simulink model "MFTiresLongitudinalSSC"  (R2026b)
settings: Solver=VariableStepAuto
undefined symbols (not defined in the file): AxlFL, AxlFR, AxlRL, AxlRR, PlntWhlDampCoeffFrnt, PlntWhlDampCoeffRear, PlntWhlLdRadius
libraries: fl_lib x16, nesl_utility_internal x10, sdl_lib x4
settings Model: Creator=The MathWorks, Inc.  LastModifiedBy=The MathWorks, Inc.
settings OptimizationCC: ReuseModelBlockBuffer=off
settings DebuggingCC: SubsystemReferenceDiagnosticForUnitTest=warning
settings SimscapeCC: SimscapeUseEnergyAccounting=off

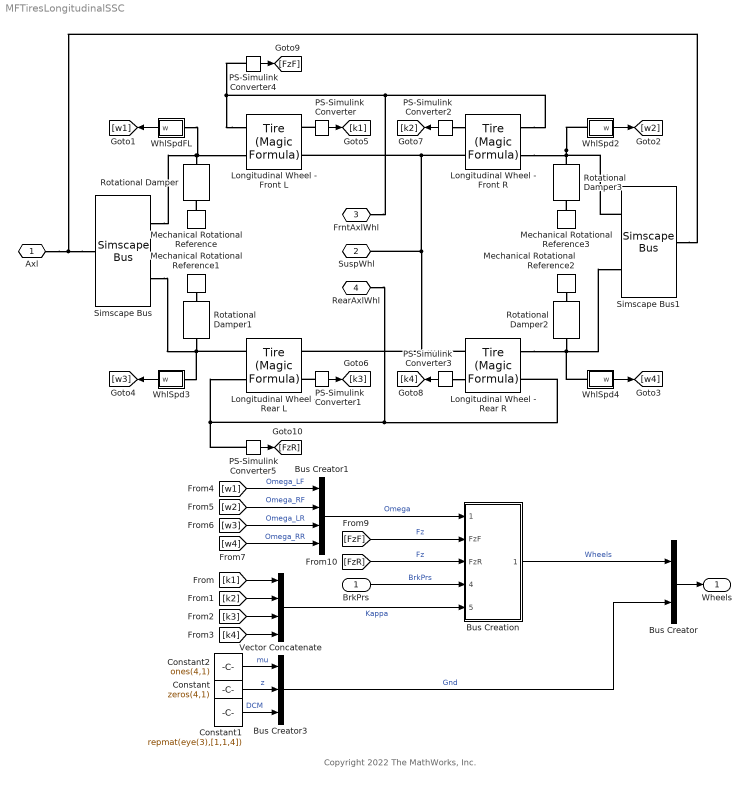
== system MFTiresLongitudinalSSC ==
  note: Copyright 2022 The MathWorks, Inc.
  BrkPrs : Inport
  Bus Creator : BusCreator  Inputs=2
  Bus Creator1 : BusCreator  Inputs=4
  Bus Creator3 : BusCreator  Inputs=3
  Bus Creation : Subsystem
  Constant : Constant  Value=zeros(4,1)  SampleTime=-1
  Constant1 : Constant  Value=repmat(eye(3),[1,1,4])  SampleTime=-1
  Constant2 : Constant  Value=ones(4,1)  SampleTime=-1
  Longitudinal Wheel - Front L : sdl_lib/Tires & Vehicles/Tire (Magic Formula)  parameterization=sdl.enum.magic_tire_model.constant  F_z1=3000 N  F_x1=3500 N  kappa1=10  B_m=PlntWhlLongStfFctr  C_m=PlntWhlLongShapeFctr  D_m=PlntWhlLongPeakFctr  E_m=PlntWhlLongCuvFctr  fz0=4000 N  p_Cx=1.685  p_Dx=[1.21, -.037]  p_Ex=[.344, .095, -.02, 0]  p_Kx=[21.51, -.163, .245]  p_Hx=[-.002, .002]  p_Vx=[0, 0]  rolling_radius_model=sdl.enum.RollingRadiusParameterization.Constant  r_e=PlntWhlLdRadius m  r_0=0.3 m  breff=8.39  dreff=0.26  freff=0.074  q_re0=0.99  q_v1=0.008  longvl=17 m/s  cz=5e5 N/m  model_resistance=simscape.enum.onoff.on  resistance_model=sdl.enum.rollingResistanceParameterization.velocity  coeff=0.015  p_tire=PlntWhlPrsFrnt Pa  alpha=PlntWhlTirPrsExp  beta=PlntWhlNrmlForceExp  coeff_a=PlntWhlVelIndpntForceCff  coeff_b=PlntWhlLnrVelForceComp s/m  coeff_c=PlntWhlQuadVelForceComp s^2/m^2  p_tire0=240e3 Pa  fz0_resistance=4000 N  vH0=16 m/s  q_Sy=[.0082, 0, .0014, .001, 0, 0, 1.08, -.5]  v_thr=PlntWhlRollResVelThresh m/s  enable_scaling_coefficients=false  lfzO=1  lcx=1  lmux=1  lex=1  lkx=1  lhx=1  lvx=1  lmy=1  model_compliance=sdl.enum.compliance.off  stiffness=PlntWhlCompStiff N/m  damping=PlntWhlCompDamp N*s/m  model_inertia=sdl.enum.model_inertia.on  inertia=PlntWhlInertiaFrnt kg*m^2  initial_velocity=0 rad/s  vxlow=1 m/s  v_tr_thr=PlntWhlVelThresh m/s  kpumin=PlntWhlMinSlipRatio  kpumax=PlntWhlMaxSlipRatio
  Longitudinal Wheel - Front R : sdl_lib/Tires & Vehicles/Tire (Magic Formula)  parameterization=sdl.enum.magic_tire_model.constant  F_z1=3000 N  F_x1=3500 N  kappa1=10  B_m=PlntWhlLongStfFctr  C_m=PlntWhlLongShapeFctr  D_m=PlntWhlLongPeakFctr  E_m=PlntWhlLongCuvFctr  fz0=4000 N  p_Cx=1.685  p_Dx=[1.21, -.037]  p_Ex=[.344, .095, -.02, 0]  p_Kx=[21.51, -.163, .245]  p_Hx=[-.002, .002]  p_Vx=[0, 0]  rolling_radius_model=sdl.enum.RollingRadiusParameterization.Constant  r_e=PlntWhlLdRadius m  r_0=0.3 m  breff=8.39  dreff=0.26  freff=0.074  q_re0=0.99  q_v1=0.008  longvl=17 m/s  cz=5e5 N/m  model_resistance=simscape.enum.onoff.on  resistance_model=sdl.enum.rollingResistanceParameterization.velocity  coeff=0.015  p_tire=PlntWhlPrsFrnt Pa  alpha=PlntWhlTirPrsExp  beta=PlntWhlNrmlForceExp  coeff_a=PlntWhlVelIndpntForceCff  coeff_b=PlntWhlLnrVelForceComp s/m  coeff_c=PlntWhlQuadVelForceComp s^2/m^2  p_tire0=240e3 Pa  fz0_resistance=4000 N  vH0=16 m/s  q_Sy=[.0082, 0, .0014, .001, 0, 0, 1.08, -.5]  v_thr=PlntWhlRollResVelThresh m/s  enable_scaling_coefficients=false  lfzO=1  lcx=1  lmux=1  lex=1  lkx=1  lhx=1  lvx=1  lmy=1  model_compliance=sdl.enum.compliance.off  stiffness=PlntWhlCompStiff N/m  damping=PlntWhlCompDamp N*s/m  model_inertia=sdl.enum.model_inertia.on  inertia=PlntWhlInertiaFrnt kg*m^2  initial_velocity=0 rad/s  vxlow=1 m/s  v_tr_thr=PlntWhlVelThresh m/s  kpumin=PlntWhlMinSlipRatio  kpumax=PlntWhlMaxSlipRatio
  Longitudinal Wheel - Rear L : sdl_lib/Tires & Vehicles/Tire (Magic Formula)  parameterization=sdl.enum.magic_tire_model.constant  F_z1=3000 N  F_x1=3500 N  kappa1=10  B_m=PlntWhlLongStfFctr  C_m=PlntWhlLongShapeFctr  D_m=PlntWhlLongPeakFctr  E_m=PlntWhlLongCuvFctr  fz0=4000 N  p_Cx=1.685  p_Dx=[1.21, -.037]  p_Ex=[.344, .095, -.02, 0]  p_Kx=[21.51, -.163, .245]  p_Hx=[-.002, .002]  p_Vx=[0, 0]  rolling_radius_model=sdl.enum.RollingRadiusParameterization.Constant  r_e=PlntWhlLdRadius m  r_0=0.3 m  breff=8.39  dreff=0.26  freff=0.074  q_re0=0.99  q_v1=0.008  longvl=17 m/s  cz=5e5 N/m  model_resistance=simscape.enum.onoff.on  resistance_model=sdl.enum.rollingResistanceParameterization.velocity  coeff=0.015  p_tire=PlntWhlPrsRear Pa  alpha=PlntWhlTirPrsExp  beta=PlntWhlNrmlForceExp  coeff_a=PlntWhlVelIndpntForceCff  coeff_b=PlntWhlLnrVelForceComp s/m  coeff_c=PlntWhlQuadVelForceComp s^2/m^2  p_tire0=240e3 Pa  fz0_resistance=4000 N  vH0=16 m/s  q_Sy=[.0082, 0, .0014, .001, 0, 0, 1.08, -.5]  v_thr=PlntWhlRollResVelThresh m/s  enable_scaling_coefficients=false  lfzO=1  lcx=1  lmux=1  lex=1  lkx=1  lhx=1  lvx=1  lmy=1  model_compliance=sdl.enum.compliance.off  stiffness=PlntWhlCompStiff N/m  damping=PlntWhlCompDamp N*s/m  model_inertia=sdl.enum.model_inertia.on  inertia=PlntWhlInertiaRear kg*m^2  initial_velocity=0 rad/s  vxlow=1 m/s  v_tr_thr=PlntWhlVelThresh m/s  kpumin=PlntWhlMinSlipRatio  kpumax=PlntWhlMaxSlipRatio
  Longitudinal Wheel - Rear R : sdl_lib/Tires & Vehicles/Tire (Magic Formula)  parameterization=sdl.enum.magic_tire_model.constant  F_z1=3000 N  F_x1=3500 N  kappa1=10  B_m=PlntWhlLongStfFctr  C_m=PlntWhlLongShapeFctr  D_m=PlntWhlLongPeakFctr  E_m=PlntWhlLongCuvFctr  fz0=4000 N  p_Cx=1.685  p_Dx=[1.21, -.037]  p_Ex=[.344, .095, -.02, 0]  p_Kx=[21.51, -.163, .245]  p_Hx=[-.002, .002]  p_Vx=[0, 0]  rolling_radius_model=sdl.enum.RollingRadiusParameterization.Constant  r_e=PlntWhlLdRadius m  r_0=0.3 m  breff=8.39  dreff=0.26  freff=0.074  q_re0=0.99  q_v1=0.008  longvl=17 m/s  cz=5e5 N/m  model_resistance=simscape.enum.onoff.on  resistance_model=sdl.enum.rollingResistanceParameterization.velocity  coeff=0.015  p_tire=PlntWhlPrsRear Pa  alpha=PlntWhlTirPrsExp  beta=PlntWhlNrmlForceExp  coeff_a=PlntWhlVelIndpntForceCff  coeff_b=PlntWhlLnrVelForceComp s/m  coeff_c=PlntWhlQuadVelForceComp s^2/m^2  p_tire0=240e3 Pa  fz0_resistance=4000 N  vH0=16 m/s  q_Sy=[.0082, 0, .0014, .001, 0, 0, 1.08, -.5]  v_thr=PlntWhlRollResVelThresh m/s  enable_scaling_coefficients=false  lfzO=1  lcx=1  lmux=1  lex=1  lkx=1  lhx=1  lvx=1  lmy=1  model_compliance=sdl.enum.compliance.off  stiffness=PlntWhlCompStiff N/m  damping=PlntWhlCompDamp N*s/m  model_inertia=sdl.enum.model_inertia.on  inertia=PlntWhlInertiaRear kg*m^2  initial_velocity=0 rad/s  vxlow=1 m/s  v_tr_thr=PlntWhlVelThresh m/s  kpumin=PlntWhlMinSlipRatio  kpumax=PlntWhlMaxSlipRatio
  Mechanical Rotational Reference{,1..3} (4 alike) : fl_lib/Mechanical/Rotational Elements/Mechanical Rotational Reference
  PS-Simulink Converter{,1..5} (6 alike) : nesl_utility_internal/PS-Simulink Converter  PhysicalDomain=network_engine_domain  SubClassName=ps_output  LeftPortType=input  RightPortType=output  PseudoPeriodic=off  Frequencies=[]  VectorFormat=inherit  Unit=inherit  AffineConversion=off
  Rotational Damper : fl_lib/Mechanical/Rotational Elements/Rotational Damper  D=PlntWhlDampCoeffFrnt N*m*s/rad  w_specify=off  w_priority=None  w=0 rad/s  w_nominal_specify=off  w_nominal_value=1  w_nominal_unit=rad/s  t_specify=off  t_priority=None  t=0 N*m  t_nominal_specify=off  t_nominal_value=1  t_nominal_unit=N*m
  Rotational Damper1 : fl_lib/Mechanical/Rotational Elements/Rotational Damper  D=PlntWhlDampCoeffRear N*m*s/rad  w_specify=off  w_priority=None  w=0 rad/s  w_nominal_specify=off  w_nominal_value=1  w_nominal_unit=rad/s  t_specify=off  t_priority=None  t=0 N*m  t_nominal_specify=off  t_nominal_value=1  t_nominal_unit=N*m
  Rotational Damper2 : fl_lib/Mechanical/Rotational Elements/Rotational Damper  D=PlntWhlDampCoeffRear N*m*s/rad  w_specify=off  w_priority=None  w=0 rad/s  w_nominal_specify=off  w_nominal_value=1  w_nominal_unit=rad/s  t_specify=off  t_priority=None  t=0 N*m  t_nominal_specify=off  t_nominal_value=1  t_nominal_unit=N*m
  Rotational Damper3 : fl_lib/Mechanical/Rotational Elements/Rotational Damper  D=PlntWhlDampCoeffFrnt N*m*s/rad  w_specify=off  w_priority=None  w=0 rad/s  w_nominal_specify=off  w_nominal_value=1  w_nominal_unit=rad/s  t_specify=off  t_priority=None  t=0 N*m  t_nominal_specify=off  t_nominal_value=1  t_nominal_unit=N*m
  Simscape Bus : SimscapeBus  HierarchyStrings=AxlFL;AxlRL
  Simscape Bus1 : SimscapeBus  HierarchyStrings=AxlFR;AxlRR
  Vector Concatenate : Concatenate  NumInputs=4
  WhlSpd2 : Subsystem
  WhlSpd3 : Subsystem
  WhlSpd4 : Subsystem
  WhlSpdFL : Subsystem
  Axl : PMIOPort  Side=Left
  SuspWhl : PMIOPort  Port=2  Side=Left
  FrntAxlWhl : PMIOPort  Port=3  Side=Left
  RearAxlWhl : PMIOPort  Port=4  Side=Left
  Wheels : Outport
  wires:
  PS-Simulink Converter5/1 -> [FzR]
  [FzF] -> Bus Creation/2(FzF)  "Fz"
  PS-Simulink Converter4/1 -> [FzF]
  WhlSpdFL/1(w) -> [w1]
  [w1] -> Bus Creator1/1  "Omega_LF"
  BrkPrs/1 -> Bus Creation/4(BrkPrs)  "BrkPrs"
  [w3] -> Bus Creator1/3  "Omega_LR"
  PS-Simulink Converter1/1 -> [k3]
  WhlSpd3/1(w) -> [w3]
  [k4] -> Vector Concatenate/4
  PS-Simulink Converter/1 -> [k1]
  [w2] -> Bus Creator1/2  "Omega_RF"
  [FzR] -> Bus Creation/3(FzR)  "Fz"
  [w4] -> Bus Creator1/4  "Omega_RR"
  Bus Creator1/1 -> Bus Creation/1(Omega)  "Omega"
  PS-Simulink Converter2/1 -> [k2]
  WhlSpd4/1(w) -> [w4]
  Vector Concatenate/1 -> Bus Creation/5(Kappa)  "Kappa"
  PS-Simulink Converter3/1 -> [k4]
  [k1] -> Vector Concatenate/1
  WhlSpd2/1(w) -> [w2]
  [k3] -> Vector Concatenate/3
  [k2] -> Vector Concatenate/2
  Bus Creation/1(Wheels) -> Bus Creator/1  "Wheels"
  Constant2/1 -> Bus Creator3/1  "mu"
  Constant/1 -> Bus Creator3/2  "z"
  Constant1/1 -> Bus Creator3/3  "DCM"
  Bus Creator3/1 -> Bus Creator/2  "Gnd"
  Bus Creator/1 -> Wheels/1
  connections:
  RearAxlWhl/RConn1 -- PS-Simulink Converter5/LConn1 -- Longitudinal Wheel - Rear L/LConn1 -- Longitudinal Wheel - Rear R/LConn1
  WhlSpdFL/LConn1 -- Rotational Damper/LConn1 -- Simscape Bus/LConn1 -- Longitudinal Wheel - Front L/LConn2
  Rotational Damper2/LConn1 -- WhlSpd4/LConn1 -- Longitudinal Wheel - Rear R/LConn2 -- Simscape Bus1/LConn2
  Longitudinal Wheel - Front L/LConn1 -- Longitudinal Wheel - Front R/LConn1 -- FrntAxlWhl/RConn1 -- PS-Simulink Converter4/LConn1
  Simscape Bus/RConn1 -- Simscape Bus1/RConn1 -- Axl/RConn1
  Longitudinal Wheel - Rear L/LConn2 -- WhlSpd3/LConn1 -- Simscape Bus/LConn2 -- Rotational Damper1/LConn1
  Simscape Bus1/LConn1 -- WhlSpd2/LConn1 -- Rotational Damper3/LConn1 -- Longitudinal Wheel - Front R/LConn2
  Longitudinal Wheel - Rear R/RConn2 -- Longitudinal Wheel - Front R/RConn2 -- Longitudinal Wheel - Front L/RConn2 -- SuspWhl/RConn1 -- Longitudinal Wheel - Rear L/RConn2
  PS-Simulink Converter1/LConn1 -- Longitudinal Wheel - Rear L/RConn1
  Mechanical Rotational Reference1/LConn1 -- Rotational Damper1/RConn1
  Mechanical Rotational Reference2/LConn1 -- Rotational Damper2/RConn1
  Mechanical Rotational Reference/LConn1 -- Rotational Damper/RConn1
  PS-Simulink Converter3/LConn1 -- Longitudinal Wheel - Rear R/RConn1
  Mechanical Rotational Reference3/LConn1 -- Rotational Damper3/RConn1
  PS-Simulink Converter/LConn1 -- Longitudinal Wheel - Front L/RConn1
  PS-Simulink Converter2/LConn1 -- Longitudinal Wheel - Front R/RConn1

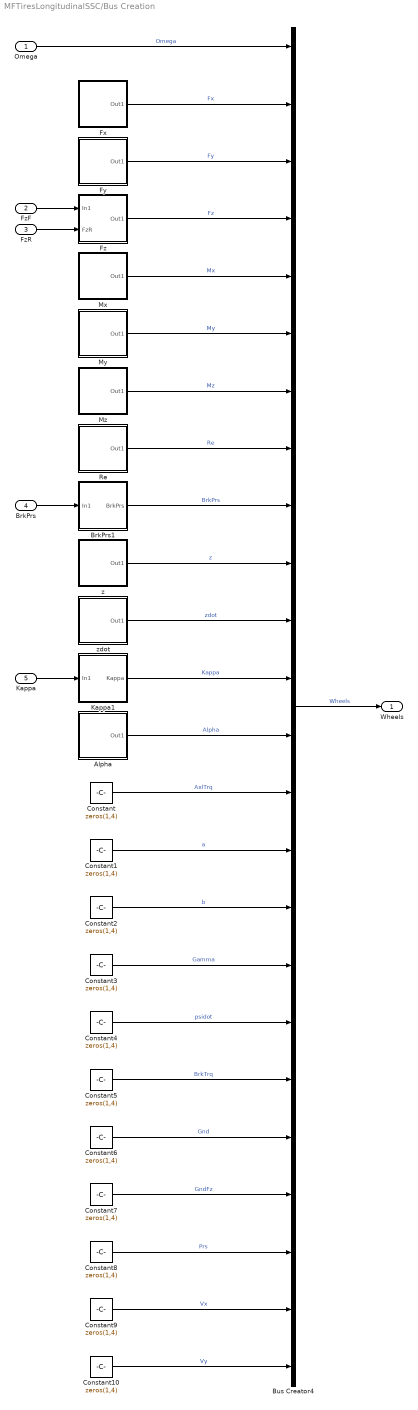
== system MFTiresLongitudinalSSC/Bus Creation ==
  Omega : Inport
  FzF : Inport  Port=2
  FzR : Inport  Port=3
  BrkPrs : Inport  Port=4
  Kappa : Inport  Port=5
  Alpha : Subsystem
  BrkPrs1 : Subsystem
  Bus Creator4 : BusCreator  Inputs=24
  Constant{,1..10} (11 alike) : Constant  Value=zeros(1,4)  SampleTime=-1
  Fx : Subsystem
  Fy : Subsystem
  Fz : Subsystem
  Kappa1 : Subsystem
  Mx : Subsystem
  My : Subsystem
  Mz : Subsystem
  Re : Subsystem
  z : Subsystem
  zdot : Subsystem
  Wheels : Outport
  wires:
  BrkPrs1/1(BrkPrs) -> Bus Creator4/9  "BrkPrs"
  Bus Creator4/1 -> Wheels/1  "Wheels"
  Alpha/1(Out1) -> Bus Creator4/13  "Alpha"
  My/1(Out1) -> Bus Creator4/6  "My"
  Fy/1(Out1) -> Bus Creator4/3  "Fy"
  z/1(Out1) -> Bus Creator4/10  "z"
  Omega/1 -> Bus Creator4/1  "Omega"
  Mz/1(Out1) -> Bus Creator4/7  "Mz"
  Kappa1/1(Kappa) -> Bus Creator4/12  "Kappa"
  zdot/1(Out1) -> Bus Creator4/11  "zdot"
  Mx/1(Out1) -> Bus Creator4/5  "Mx"
  Fx/1(Out1) -> Bus Creator4/2  "Fx"
  Fz/1(Out1) -> Bus Creator4/4  "Fz"
  Re/1(Out1) -> Bus Creator4/8  "Re"
  FzF/1 -> Fz/1(In1)
  FzR/1 -> Fz/2(FzR)
  BrkPrs/1 -> BrkPrs1/1(In1)
  Kappa/1 -> Kappa1/1(In1)
  Constant/1 -> Bus Creator4/14  "AxlTrq"
  Constant1/1 -> Bus Creator4/15  "a"
  Constant2/1 -> Bus Creator4/16  "b"
  Constant3/1 -> Bus Creator4/17  "Gamma"
  Constant4/1 -> Bus Creator4/18  "psidot"
  Constant5/1 -> Bus Creator4/19  "BrkTrq"
  Constant6/1 -> Bus Creator4/20  "Gnd"
  Constant7/1 -> Bus Creator4/21  "GndFz"
  Constant8/1 -> Bus Creator4/22  "Prs"
  Constant9/1 -> Bus Creator4/23  "Vx"
  Constant10/1 -> Bus Creator4/24  "Vy"

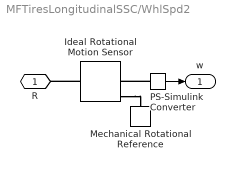
== system MFTiresLongitudinalSSC/WhlSpd2 ==
  Ideal Rotational Motion Sensor : fl_lib/Mechanical/Mechanical Sensors/Ideal Rotational Motion Sensor  reference=foundation.enum.MeasurementReference.difference  acceleration_port=false  velocity_port=true  position_port=true  wrap_angle=simscape.enum.onoff.off  offset=0 rad
  Mechanical Rotational Reference : fl_lib/Mechanical/Rotational Elements/Mechanical Rotational Reference
  PS-Simulink Converter : nesl_utility_internal/PS-Simulink Converter  PhysicalDomain=network_engine_domain  SubClassName=ps_output  LeftPortType=input  RightPortType=output  PseudoPeriodic=off  Frequencies=[]  VectorFormat=inherit  Unit=inherit  AffineConversion=off
  R : PMIOPort  Side=Left
  w : Outport
  wires:
  PS-Simulink Converter/1 -> w/1
  connections:
  PS-Simulink Converter/LConn1 -- Ideal Rotational Motion Sensor/RConn2
  Ideal Rotational Motion Sensor/LConn1 -- R/RConn1
  Ideal Rotational Motion Sensor/RConn1 -- Mechanical Rotational Reference/LConn1

== system MFTiresLongitudinalSSC/WhlSpd3 ==
  Ideal Rotational Motion Sensor : fl_lib/Mechanical/Mechanical Sensors/Ideal Rotational Motion Sensor  reference=foundation.enum.MeasurementReference.difference  acceleration_port=false  velocity_port=true  position_port=true  wrap_angle=simscape.enum.onoff.off  offset=0 rad
  Mechanical Rotational Reference : fl_lib/Mechanical/Rotational Elements/Mechanical Rotational Reference
  PS-Simulink Converter : nesl_utility_internal/PS-Simulink Converter  PhysicalDomain=network_engine_domain  SubClassName=ps_output  LeftPortType=input  RightPortType=output  PseudoPeriodic=off  Frequencies=[]  VectorFormat=inherit  Unit=inherit  AffineConversion=off
  R : PMIOPort  Side=Left
  w : Outport
  wires:
  PS-Simulink Converter/1 -> w/1
  connections:
  PS-Simulink Converter/LConn1 -- Ideal Rotational Motion Sensor/RConn2
  Ideal Rotational Motion Sensor/LConn1 -- R/RConn1
  Ideal Rotational Motion Sensor/RConn1 -- Mechanical Rotational Reference/LConn1

== system MFTiresLongitudinalSSC/WhlSpd4 ==
  Ideal Rotational Motion Sensor : fl_lib/Mechanical/Mechanical Sensors/Ideal Rotational Motion Sensor  reference=foundation.enum.MeasurementReference.difference  acceleration_port=false  velocity_port=true  position_port=true  wrap_angle=simscape.enum.onoff.off  offset=0 rad
  Mechanical Rotational Reference : fl_lib/Mechanical/Rotational Elements/Mechanical Rotational Reference
  PS-Simulink Converter : nesl_utility_internal/PS-Simulink Converter  PhysicalDomain=network_engine_domain  SubClassName=ps_output  LeftPortType=input  RightPortType=output  PseudoPeriodic=off  Frequencies=[]  VectorFormat=inherit  Unit=inherit  AffineConversion=off
  R : PMIOPort  Side=Left
  w : Outport
  wires:
  PS-Simulink Converter/1 -> w/1
  connections:
  Ideal Rotational Motion Sensor/RConn1 -- Mechanical Rotational Reference/LConn1
  Ideal Rotational Motion Sensor/LConn1 -- R/RConn1
  PS-Simulink Converter/LConn1 -- Ideal Rotational Motion Sensor/RConn2

== system MFTiresLongitudinalSSC/WhlSpdFL ==
  Ideal Rotational Motion Sensor : fl_lib/Mechanical/Mechanical Sensors/Ideal Rotational Motion Sensor  reference=foundation.enum.MeasurementReference.difference  acceleration_port=false  velocity_port=true  position_port=true  wrap_angle=simscape.enum.onoff.off  offset=0 rad
  Mechanical Rotational Reference : fl_lib/Mechanical/Rotational Elements/Mechanical Rotational Reference
  PS-Simulink Converter : nesl_utility_internal/PS-Simulink Converter  PhysicalDomain=network_engine_domain  SubClassName=ps_output  LeftPortType=input  RightPortType=output  PseudoPeriodic=off  Frequencies=[]  VectorFormat=inherit  Unit=inherit  AffineConversion=off
  R : PMIOPort  Side=Left
  w : Outport
  wires:
  PS-Simulink Converter/1 -> w/1
  connections:
  Ideal Rotational Motion Sensor/RConn1 -- Mechanical Rotational Reference/LConn1
  Ideal Rotational Motion Sensor/LConn1 -- R/RConn1
  PS-Simulink Converter/LConn1 -- Ideal Rotational Motion Sensor/RConn2

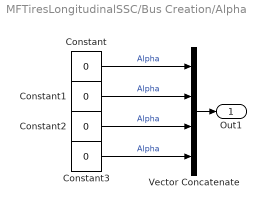
== system MFTiresLongitudinalSSC/Bus Creation/Alpha ==
  Constant{,1..3} (4 alike) : Constant  Value=0  SampleTime=-1
  Vector Concatenate : Concatenate  NumInputs=4
  Out1 : Outport  VectorParamsAs1DForOutWhenUnconnected=off
  wires:
  Constant2/1 -> Vector Concatenate/3  "Alpha"
  Constant3/1 -> Vector Concatenate/4  "Alpha"
  Constant/1 -> Vector Concatenate/1  "Alpha"
  Constant1/1 -> Vector Concatenate/2  "Alpha"
  Vector Concatenate/1 -> Out1/1

== system MFTiresLongitudinalSSC/Bus Creation/BrkPrs1 ==
  In1 : Inport
  BrkPrs : Outport  VectorParamsAs1DForOutWhenUnconnected=off
  wires:
  In1/1 -> BrkPrs/1  "BrkPrs"

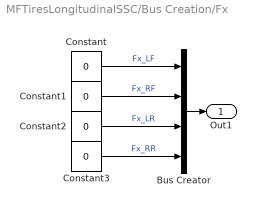
== system MFTiresLongitudinalSSC/Bus Creation/Fx ==
  Bus Creator : BusCreator  Inputs=4
  Constant{,1..3} (4 alike) : Constant  Value=0  SampleTime=-1
  Out1 : Outport  VectorParamsAs1DForOutWhenUnconnected=off
  wires:
  Constant3/1 -> Bus Creator/4  "Fx_RR"
  Constant2/1 -> Bus Creator/3  "Fx_LR"
  Constant1/1 -> Bus Creator/2  "Fx_RF"
  Constant/1 -> Bus Creator/1  "Fx_LF"
  Bus Creator/1 -> Out1/1

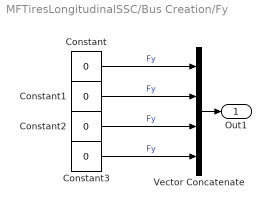
== system MFTiresLongitudinalSSC/Bus Creation/Fy ==
  Constant{,1..3} (4 alike) : Constant  Value=0  SampleTime=-1
  Vector Concatenate : Concatenate  NumInputs=4
  Out1 : Outport  VectorParamsAs1DForOutWhenUnconnected=off
  wires:
  Constant3/1 -> Vector Concatenate/4  "Fy"
  Constant2/1 -> Vector Concatenate/3  "Fy"
  Constant1/1 -> Vector Concatenate/2  "Fy"
  Vector Concatenate/1 -> Out1/1
  Constant/1 -> Vector Concatenate/1  "Fy"

== system MFTiresLongitudinalSSC/Bus Creation/Fz ==
  In1 : Inport
  FzR : Inport  Port=2
  Vector Concatenate : Concatenate  NumInputs=4
  Out1 : Outport  VectorParamsAs1DForOutWhenUnconnected=off
  wires:
  Vector Concatenate/1 -> Out1/1
  In1/1 -> Vector Concatenate/2, Vector Concatenate/1
  FzR/1 -> Vector Concatenate/4, Vector Concatenate/3

== system MFTiresLongitudinalSSC/Bus Creation/Kappa1 ==
  In1 : Inport
  Kappa : Outport  VectorParamsAs1DForOutWhenUnconnected=off
  wires:
  In1/1 -> Kappa/1  "Kappa"

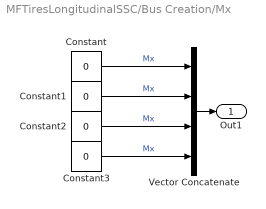
== system MFTiresLongitudinalSSC/Bus Creation/Mx ==
  Constant{,1..3} (4 alike) : Constant  Value=0  SampleTime=-1
  Vector Concatenate : Concatenate  NumInputs=4
  Out1 : Outport  VectorParamsAs1DForOutWhenUnconnected=off
  wires:
  Constant2/1 -> Vector Concatenate/3  "Mx"
  Constant3/1 -> Vector Concatenate/4  "Mx"
  Constant/1 -> Vector Concatenate/1  "Mx"
  Constant1/1 -> Vector Concatenate/2  "Mx"
  Vector Concatenate/1 -> Out1/1

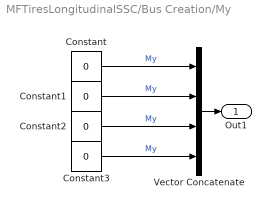
== system MFTiresLongitudinalSSC/Bus Creation/My ==
  Constant{,1..3} (4 alike) : Constant  Value=0  SampleTime=-1
  Vector Concatenate : Concatenate  NumInputs=4
  Out1 : Outport  VectorParamsAs1DForOutWhenUnconnected=off
  wires:
  Vector Concatenate/1 -> Out1/1
  Constant/1 -> Vector Concatenate/1  "My"
  Constant1/1 -> Vector Concatenate/2  "My"
  Constant2/1 -> Vector Concatenate/3  "My"
  Constant3/1 -> Vector Concatenate/4  "My"

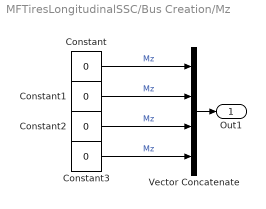
== system MFTiresLongitudinalSSC/Bus Creation/Mz ==
  Constant{,1..3} (4 alike) : Constant  Value=0  SampleTime=-1
  Vector Concatenate : Concatenate  NumInputs=4
  Out1 : Outport  VectorParamsAs1DForOutWhenUnconnected=off
  wires:
  Constant2/1 -> Vector Concatenate/3  "Mz"
  Constant3/1 -> Vector Concatenate/4  "Mz"
  Constant/1 -> Vector Concatenate/1  "Mz"
  Constant1/1 -> Vector Concatenate/2  "Mz"
  Vector Concatenate/1 -> Out1/1

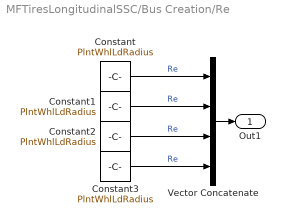
== system MFTiresLongitudinalSSC/Bus Creation/Re ==
  Constant{,1..3} (4 alike) : Constant  Value=PlntWhlLdRadius  SampleTime=-1
  Vector Concatenate : Concatenate  NumInputs=4
  Out1 : Outport  VectorParamsAs1DForOutWhenUnconnected=off
  wires:
  Vector Concatenate/1 -> Out1/1
  Constant/1 -> Vector Concatenate/1  "Re"
  Constant1/1 -> Vector Concatenate/2  "Re"
  Constant2/1 -> Vector Concatenate/3  "Re"
  Constant3/1 -> Vector Concatenate/4  "Re"

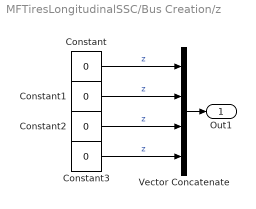
== system MFTiresLongitudinalSSC/Bus Creation/z ==
  Constant{,1..3} (4 alike) : Constant  Value=0  SampleTime=-1
  Vector Concatenate : Concatenate  NumInputs=4
  Out1 : Outport  VectorParamsAs1DForOutWhenUnconnected=off
  wires:
  Constant3/1 -> Vector Concatenate/4  "z"
  Constant2/1 -> Vector Concatenate/3  "z"
  Constant1/1 -> Vector Concatenate/2  "z"
  Constant/1 -> Vector Concatenate/1  "z"
  Vector Concatenate/1 -> Out1/1

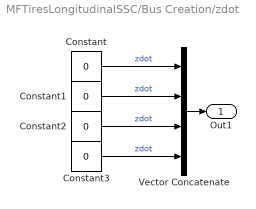
== system MFTiresLongitudinalSSC/Bus Creation/zdot ==
  Constant{,1..3} (4 alike) : Constant  Value=0  SampleTime=-1
  Vector Concatenate : Concatenate  NumInputs=4
  Out1 : Outport  VectorParamsAs1DForOutWhenUnconnected=off
  wires:
  Vector Concatenate/1 -> Out1/1
  Constant/1 -> Vector Concatenate/1  "zdot"
  Constant1/1 -> Vector Concatenate/2  "zdot"
  Constant2/1 -> Vector Concatenate/3  "zdot"
  Constant3/1 -> Vector Concatenate/4  "zdot"
